simulink model "DCmotorArduinoUno"  (R2021b)
settings: Solver=FixedStepAuto  StartTime=0.0  StopTime=inf  FixedStep=.005  RelTol=1e-3  EnableMultiTasking=on
InitFcn:
  | pos = 0;
  | vel = 0;
model workspace: external: MATLAB File C:\My_Disk\work\school\grad\ME5245\finalProject\simulinkParameters.m (data not in the file)
values from neighbouring files (symbols this model uses):
  J = 0.018256    [simulinkParameters.m]
  Ts = 0.05    [simulinkParameters.m]
undefined symbols (not defined in the file or in its folder): DiscIntNeverNeededParam
libraries: arduinolib x8, fl_lib x5, nesl_utility x5, ee_lib x2, arduinosensorlib x1, slpidlib x1, simulink x1
settings Model: ExtModeTrigDuration=2  Creator=min  LastModifiedBy=min
settings SolverCC: PositivePriorityOrder=on  AutoInsertRateTranBlk=on  MinimalZcImpactIntegration=on
settings OptimizationCC: EnhancedBackFolding=on  PassReuseOutputArgsAs=Individual arguments  ZeroExternalMemoryAtStartup=off  ZeroInternalMemoryAtStartup=off  MaxStackSize=64  OptimizeBlockOrder=speed  DifferentSizesBufferReuse=on  OptimizationCustomize=off  EfficientTunableParamExpr=on
settings DebuggingCC: ReadBeforeWriteMsg=DisableAll  WriteAfterWriteMsg=DisableAll  WriteAfterReadMsg=DisableAll  TasksWithSamePriorityMsg=none  ParameterTunabilityLossMsg=error
settings HardwareCC: ProdBitPerInt=16  ProdBitPerPointer=16  ProdBitPerSizeT=16  ProdBitPerPtrDiffT=16  ProdLargestAtomicFloat=None  ProdWordSize=8  ProdHWDeviceType=Atmel->AVR  UseEmbeddedCoderFeatures=off
settings ModelReferenceCC: UpdateModelReferenceTargets=IfOutOfDate
settings SFSimCC: SFSimEcho=off  MATLABDynamicMemAlloc=off
settings RTWCC: Description=Embedded Coder  SystemTargetFile=ert.tlc  HardwareBoard=Arduino Uno  TemplateMakefile=ert_default_tmf  Toolchain=Arduino AVR  BuildConfiguration=Faster Runs  CodeExecutionProfiling=on  TargetLang=C++
settings CodeAppCC: ForceParamTrailComments=on  IgnoreCustomStorageClasses=off  OperatorAnnotations=on  SimulinkDataObjDesc=on  SFDataObjDesc=on  InsertBlockDesc=on
settings ERTTargetCC: CodeInterfacePackaging=C++ class  SupportContinuousTime=on  SupportNonInlinedSFcns=on  SupportVariableSizeSignals=on  ExtModeTransport=3  ExtModeStaticAlloc=on  ExtModeStaticAllocSize=250  ExtModeMexFile=ext_xcp  ExtModeIntrfLevel=Level2 - Open  RootIOFormat=Structure reference

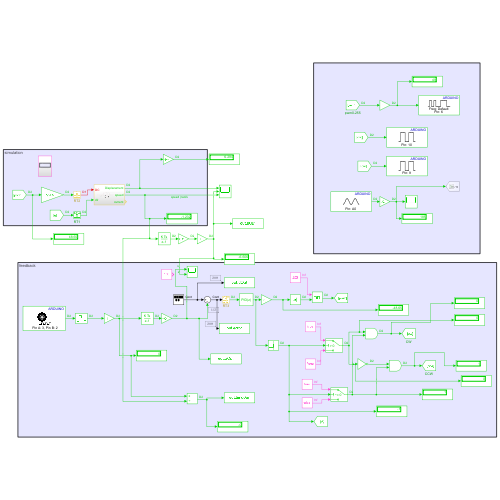
[thumbnail: Simulink's stored preview of the top-level diagram]
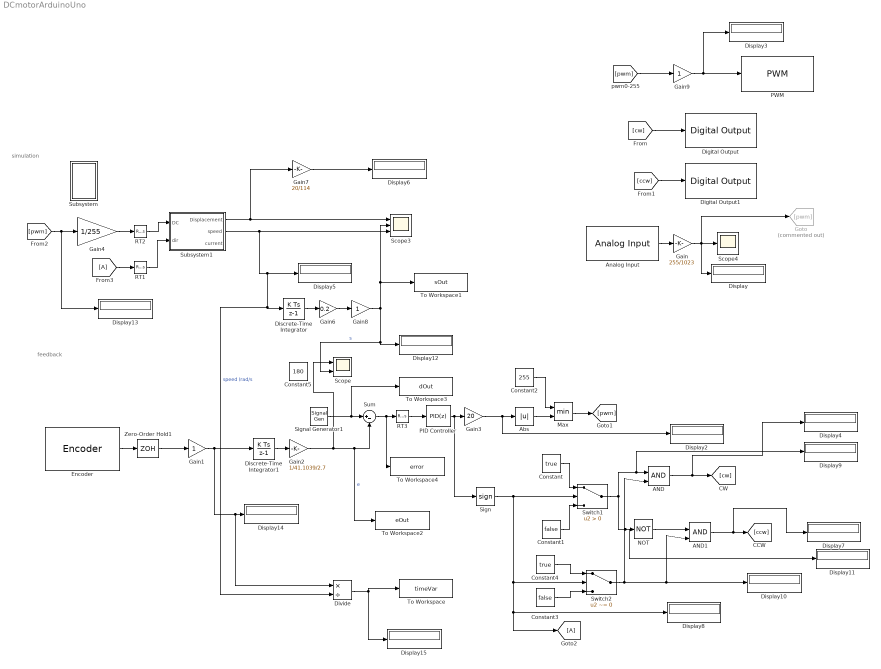
== system DCmotorArduinoUno ==
  note: feedback
  note: simulation
  AND : Logic  IconShape=distinctive  AllPortsSameDT=off  OutDataTypeStr=boolean
  AND1 : Logic  IconShape=distinctive  AllPortsSameDT=off  OutDataTypeStr=boolean
  Abs : Abs
  Analog Input : arduinolib/Analog Input  pinNumber=0  ReadResultsOnly=off  ConversionTriggerSource=Software  ExternalTriggerType=uint32( 0 )  OutputDataType=uint16  EnableConversionCompleteNotify=off  EnableOuputStatus=off  SampleTime=Ts  blockPlatform=arduino
  Constant : Constant  Value=true
  Constant1 : Constant  Value=false
  Constant2 : Constant  Value=255
  Constant3 : Constant  Value=false
  Constant4 : Constant  Value=true
  Constant5 : Constant  Value=180
  Digital Output : arduinolib/Digital Output  pinNumber=driverIn1pin  Direction=output  blockPlatform=arduino
  Digital Output1 : arduinolib/Digital Output  pinNumber=driverIn2pin  Direction=output  blockPlatform=arduino
  Discrete-Time Integrator : DiscreteIntegrator  SampleTime=-1  ICPrevOutput=DiscIntNeverNeededParam  ICPrevScaledInput=DiscIntNeverNeededParam
  Discrete-Time Integrator1 : DiscreteIntegrator  SampleTime=-1  ICPrevOutput=DiscIntNeverNeededParam  ICPrevScaledInput=DiscIntNeverNeededParam
  Display{,2..15} (15 alike) : Display
  Divide : Product  Inputs=*/
  Encoder : arduinosensorlib/Encoder  InputA=3  InputB=2  Mode=Reset at each Sample time  SampleTime=Ts
      settings: SourceProductBaseCode=ARDUINO
  Gain : Gain  Gain=255/1023  OutDataTypeStr=uint8  RndMeth=Nearest
  Gain1 : Gain  OutDataTypeStr=int32
  Gain2 : Gain  Gain=1/41.1039/2.7
  Gain3 : Gain  Gain=20
  Gain4 : Gain  Gain=1/255  OutDataTypeStr=double
  Gain6 : Gain  Gain=0.2
  Gain7 : Gain  Gain=20/114
  Gain8 : Gain
  Gain9 : Gain  OutDataTypeStr=uint8  RndMeth=Nearest
  Goto : Goto  Commented=on  GotoTag=pwm
  Max : MinMax  Inputs=2
  NOT : Logic  Operator=NOT  IconShape=distinctive  AllPortsSameDT=off  OutDataTypeStr=boolean
  PID Controller : slpidlib/PID Controller  Controller=PID  Form=Parallel  TimeDomain=Discrete-time  UseExternalTs=off  SampleTime=-1  IntegratorMethod=Forward Euler  FilterMethod=Forward Euler  ControllerParametersSource=internal  P=.12  I=.71  D=0  UseFilter=on  N=100  TunerSelectOption=Transfer Function Based (PID Tuner App)  InitialConditionSource=internal  InitialConditionForIntegrator=0  InitialConditionForFilter=0  DifferentiatorICPrevScaledInput=0  ExternalReset=none  TrackingMode=off  Kt=1  LimitOutput=off  SatLimitsSource=internal  UpperSaturationLimit=inf  LowerSaturationLimit=-inf  LinearizeAsGain=on  AntiWindupMode=none  Kb=1  POutMin=[]  POutMax=[]  IOutMin=[]  IOutMax=[]  DOutMin=[]  DOutMax=[]  NOutMin=[]  NOutMax=[]  SumOutMin=[]  SumOutMax=[]  SaturationOutMin=[]  SaturationOutMax=[]  PParamMin=[]  PParamMax=[]  IParamMin=[]  IParamMax=[]  DParamMin=[]  DParamMax=[]  NParamMin=[]  NParamMax=[]  KbParamMin=[]  KbParamMax=[]  KtParamMin=[]  KtParamMax=[]  KbOutMin=[]  KbOutMax=[]  KtOutMin=[]  KtOutMax=[]  IntegratorOutMin=[]  IntegratorOutMax=[]  FilterOutMin=[]  FilterOutMax=[]  SumI1OutMin=[]  SumI1OutMax=[]  SumI2OutMin=[]  SumI2OutMax=[]  SumI3OutMin=[]  SumI3OutMax=[]  SumI4OutMin=[]  SumI4OutMax=[]  SumDOutMin=[]  SumDOutMax=[]  DifferentiatorOutMin=[]  DifferentiatorOutMax=[]  FilterDiffOutCoefMin=[]  FilterDiffOutCoefMax=[]  ReciprocalOutMin=[]  ReciprocalOutMax=[]  SumDenOutMin=[]  SumDenOutMax=[]  SumNumOutMin=[]  SumNumOutMax=[]  DivideOutMin=[]  DivideOutMax=[]  UdiffTsProdOutMin=[]  UdiffTsProdOutMax=[]  NTsProdOutMin=[]  NTsProdOutMax=[]  UintegralTsProdOutMin=[]  UintegralTsProdOutMax=[]  UngainTsProdOutMin=[]  UngainTsProdOutMax=[]  IntegratorContinuousStateAttributes=''  IntegratorStateMustResolveToSignalObject=off  IntegratorRTWStateStorageClass=Auto  FilterContinuousStateAttributes=''  FilterStateMustResolveToSignalObject=off  FilterRTWStateStorageClass=Auto  ParallelPVariant=InternalParameters  IdealPVariant=Disabled  IVariant=InternalParameters  DVariant=InternalParameters  IntegratorVariant=Discrete  SatVariant=Disabled  AWVariant=Passthrough  PCopyVariant=Disabled  TRVariant=Disabled  FdbkBlocksVariant=Forward  IdealPFdbkVariant=Disabled  SatFdbkVariant=Disabled  DerivativeFilterVariant=ForwardEulerFilter  NVariant=InternalParameters  NCopyVariant=Disabled  FilterICVariant=InternalICsFilter  IntegratorICVariant=InternalICs  ExternalResetVariant=Disabled  TRSumVariant=Passthrough  SumFdbkVariant=Disabled  SumVariant=Sum_PID  TsampFilterVariant=InternalTs  TsampNgainVariant=Passthrough  TsampIntegralVariant=Passthrough  ExternalSaturationOutDataTypeStr=Inherit: Same as second input
  PWM : arduinolib/PWM  pinNumber=6  frequencyType=Default  desiredFrequency=490.2  achievableFrequency=490.2
  RT1 : RateTransition  OutPortSampleTime=Ts
  RT2 : RateTransition  OutPortSampleTime=5e-3
  RT3 : RateTransition  OutPortSampleTime=Ts
  Scope : Scope  NumInputPorts=2
  Scope3 : Scope  NumInputPorts=3
  Scope4 : Scope
  Sign : Signum
  Signal Generator1 : SignalGenerator  WaveForm=square  Amplitude=pi/2  Frequency=.1
  Subsystem : Subsystem
  Subsystem1 : Subsystem
  Sum : Sum  Inputs=|+-
  Switch1 : Switch  Criteria=u2 > Threshold
  Switch2 : Switch  Criteria=u2 ~= 0
  To Workspace : ToWorkspace  VariableName=timeVar  SaveFormat=Timeseries  SampleTime=-1
  To Workspace1 : ToWorkspace  VariableName=sOut  SaveFormat=Timeseries  SampleTime=-1
  To Workspace2 : ToWorkspace  VariableName=eOut  SaveFormat=Timeseries  SampleTime=-1
  To Workspace3 : ToWorkspace  VariableName=dOut  SaveFormat=Timeseries  SampleTime=Ts
  To Workspace4 : ToWorkspace  VariableName=error  SaveFormat=Timeseries  SampleTime=Ts
  Zero-Order Hold1 : ZeroOrderHold  SampleTime=Ts
  wires:
  Analog Input/1 -> Gain/1
  Encoder/1 -> Zero-Order Hold1/1
  Zero-Order Hold1/1 -> Gain1/1
  Gain1/1 -> Discrete-Time Integrator1/1, Divide/1, Display14/1
  Gain/1 -> Display/1, Scope4/1, Goto/1
  Subsystem1/2(speed) -> Scope3/3, Divide/2, Discrete-Time Integrator/1, Display5/1  "speed (rad/s"
  RT2/1 -> Subsystem1/1(DC)
  Gain4/1 -> RT2/1
  Switch1/1 -> Display11/1, NOT/1, Display9/1, AND/1
  Constant1/1 -> Switch1/3
  Constant/1 -> Switch1/1
  Sign/1 -> Switch2/2, [A], Display8/1, Switch1/2
  Signal Generator1/1 -> To Workspace3/1, Sum/1
  Max/1 -> [pwm]
  Constant2/1 -> Max/1
  Abs/1 -> Max/2
  Switch2/1 -> AND1/2, Display10/1, AND/2
  AND/1 -> Display4/1, [cw]
  NOT/1 -> AND1/1
  AND1/1 -> Display7/1, [ccw]
  Gain3/1 -> Display2/1, Abs/1
  Constant4/1 -> Switch2/1
  Constant3/1 -> Switch2/3
  Subsystem1/1(Displacement) -> Gain7/1, Scope3/1
  Discrete-Time Integrator/1 -> Gain6/1
  [A] -> RT1/1
  Gain6/1 -> Gain8/1
  Gain7/1 -> Display6/1
  Gain8/1 -> Scope/2, Display12/1, To Workspace1/1, Scope3/2  "s"
  RT1/1 -> Subsystem1/2(dir)
  RT3/1 -> PID Controller/1
  Sum/1 -> To Workspace4/1, RT3/1
  PID Controller/1 -> Gain3/1, Sign/1
  Gain9/1 -> Display3/1, PWM/1
  [pwm] -> Gain9/1
  [cw] -> Digital Output/1
  Divide/1 -> Display15/1, To Workspace/1
  [pwm] -> Display13/1, Gain4/1
  Discrete-Time Integrator1/1 -> Gain2/1
  Gain2/1 -> To Workspace2/1, Sum/2, Scope/1  "e"
  [ccw] -> Digital Output1/1

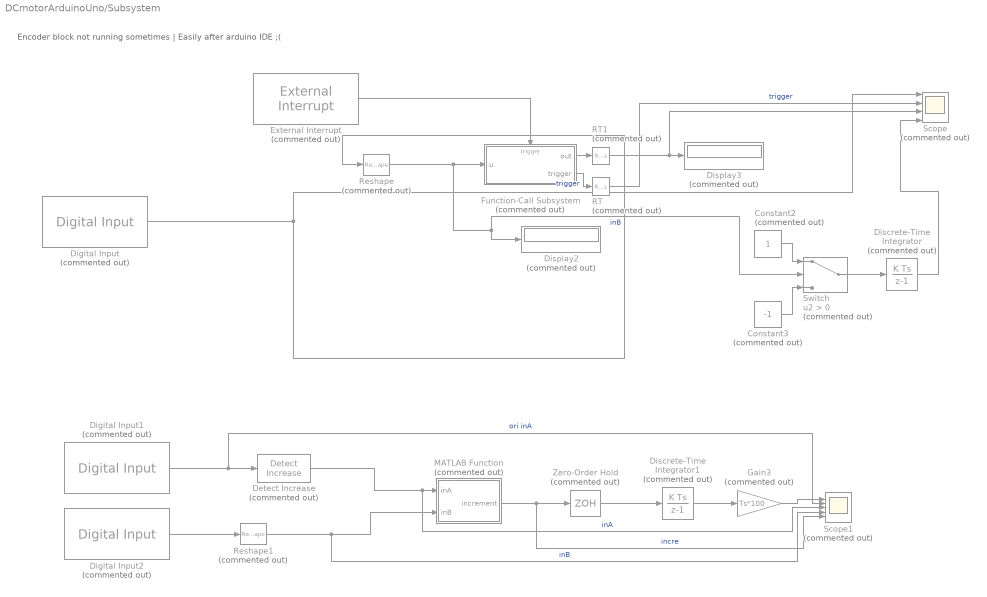
== system DCmotorArduinoUno/Subsystem ==
  note: Encoder block not running sometimes | Easily after arduino IDE ;(
  Constant2 : Constant  Commented=on
  Constant3 : Constant  Commented=on  Value=-1
  Detect Increase : simulink/Logic and Bit Operations/Detect Increase  Commented=on  vinit=0.0  OutDataTypeStr=boolean
  Digital Input : arduinolib/Digital Input  Commented=on  pinNumber=2  mode=Default  Direction=input  SampleTime=Ts  blockPlatform=arduino
  Digital Input1 : arduinolib/Digital Input  Commented=on  pinNumber=3  mode=Default  Direction=input  SampleTime=-1  blockPlatform=arduino
  Digital Input2 : arduinolib/Digital Input  Commented=on  pinNumber=2  mode=Default  Direction=input  SampleTime=Ts  blockPlatform=arduino
  Discrete-Time Integrator : DiscreteIntegrator  Commented=on  gainval=100  SampleTime=Ts  ICPrevOutput=DiscIntNeverNeededParam  ICPrevScaledInput=DiscIntNeverNeededParam
  Discrete-Time Integrator1 : DiscreteIntegrator  Commented=on  SampleTime=-1  ICPrevOutput=DiscIntNeverNeededParam  ICPrevScaledInput=DiscIntNeverNeededParam
  Display2 : Display  Commented=on
  Display3 : Display  Commented=on
  External Interrupt : arduinolib/External Interrupt  Commented=on  Pin=3  PullUp=off  Mode=RISING  InterruptSimulationInput=off
      settings: SourceProductBaseCode=ARDUINO
  Function-Call Subsystem : Subsystem  Commented=on  InitFcn=|  TreatAsAtomicUnit=on  mask{pos=pos, vel=vel}
      | pos = 0;
      | vel = 0;
      mask prompts: pos "Global Pos var"; vel "Global Vel var"
  Gain3 : Gain  Commented=on  Gain=Ts*100
  MATLAB Function : MATLAB Function  Commented=on  TreatAsAtomicUnit=on
  RT : RateTransition  Commented=on  Deterministic=off
  RT1 : RateTransition  Commented=on  Deterministic=off
  Reshape : Reshape  Commented=on
  Reshape1 : Reshape  Commented=on
  Scope : Scope  Commented=on  NumInputPorts=4
  Scope1 : Scope  Commented=on  NumInputPorts=5
  Switch : Switch  Commented=on  Criteria=u2 > Threshold
  Zero-Order Hold : ZeroOrderHold  Commented=on  SampleTime=-1
  wires:
  RT1/1 -> Display3/1, Scope/3
  Digital Input/1 -> Scope/1, Reshape/1
  Gain3/1 -> Scope1/1
  Constant2/1 -> Switch/1
  Digital Input1/1 -> Scope1/2, Detect Increase/1  "ori inA"
  Reshape/1 -> Switch/2, Display2/1, Function-Call Subsystem/1(u)  "inB"
  Zero-Order Hold/1 -> Discrete-Time Integrator1/1
  Discrete-Time Integrator1/1 -> Gain3/1
  Function-Call Subsystem/2(trigger) -> RT/1  "trigger"
  Constant3/1 -> Switch/3
  RT/1 -> Scope/2  "trigger"
  MATLAB Function/1(increment) -> Scope1/5, Zero-Order Hold/1  "incre"
  Detect Increase/1 -> Scope1/3, MATLAB Function/1(inA)  "inA"
  Function-Call Subsystem/1(out) -> RT1/1
  Discrete-Time Integrator/1 -> Scope/4
  Digital Input2/1 -> Reshape1/1
  Switch/1 -> Discrete-Time Integrator/1
  External Interrupt/1 -> Function-Call Subsystem/Trigger
  Reshape1/1 -> Scope1/4, MATLAB Function/2(inB)  "inB"

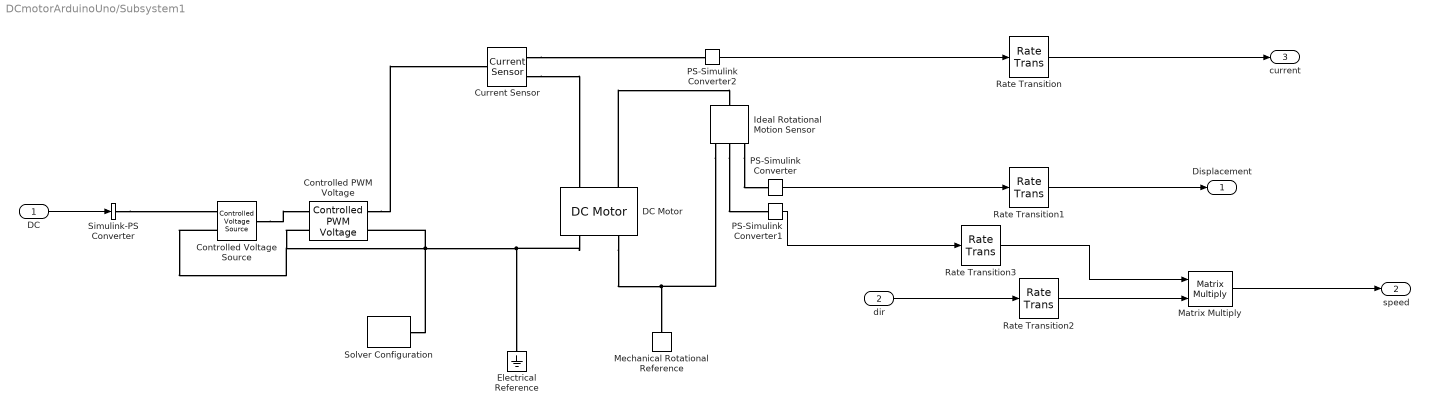
== system DCmotorArduinoUno/Subsystem1 ==
  DC : Inport
  dir : Inport  Port=2
  Controlled PWM Voltage : ee_lib/Integrated Circuits/Controlled PWM Voltage  F=100 Hz  TD=0 s  pulse_width_offset=0 s  pulse_min=0 s  pwm_or_av=1  event_type=1  sample_time=1e-6 s  Vmin=0 V  Vmax=1 V  Vm=6 V  u_min=0  u_max=1
  Controlled Voltage Source : fl_lib/Electrical/Electrical Sources/Controlled Voltage Source
  Current Sensor : fl_lib/Electrical/Electrical Sensors/Current Sensor
  DC Motor : ee_lib/Electromechanical/Brushed Motors/DC Motor  field_option=ee.enum.field_option.pm  Rf=100 Ohm  Lf=1 H  Laf=0.15 H  If0=0 A  parameterization=ee.enum.dcparam_option.circuit_param  Ra=R Ohm  La=L H  emf_or_torque=ee.enum.emf_or_torque.kv  Kv=kb V/(rad/s)  Ki=6.876e-4 N*m/A  T_stall=0.24e-3 N*m  w_max=19100 rpm  w_rated=15000 rpm  P_rated=0.08 W  V_rated=1.5 V  lam_param=ee.enum.lam_param.damping  i_noload=0 A  V_i_noload=1.5 V  J=J kg*m^2  lam=b N*m/(rad/s)  speed0=0 rpm  enable_fault_armature=simscape.enum.onoff.off  rev_faulted=1 / 3  G_faulted_armature=1e-5 S  fault_trigger_armature=ee.enum.faults.faultTrigger.temporal  t_fault_armature=1 s  max_permissible_current_armature=inf A  t_fail_on_current_armature=1 s  enable_fault_field=simscape.enum.onoff.off  G_faulted_field=1e-5 S  fault_trigger_field=ee.enum.faults.faultTrigger.temporal  t_fault_field=1 s  max_permissible_current_field=inf A  t_fail_on_current_field=1 s  fault_action=simscape.enum.assert.action.none  alpha=3.93e-3 1/K  Tmeas=25 degC  thermal_mass=100 J/K  initial_temperature=25 degC
  Electrical Reference : fl_lib/Electrical/Electrical Elements/Electrical Reference
  Ideal Rotational Motion Sensor : fl_lib/Mechanical/Mechanical Sensors/Ideal Rotational Motion Sensor  wrap_angle=simscape.enum.onoff.off  offset=0 rad
  Matrix Multiply : Product  Multiplication=Matrix(*)
  Mechanical Rotational Reference : fl_lib/Mechanical/Rotational Elements/Mechanical Rotational Reference
  PS-Simulink Converter : nesl_utility/PS-Simulink Converter  PhysicalDomain=network_engine_domain  SubClassName=ps_output  LeftPortType=input  RightPortType=output  PseudoPeriodic=off  Frequencies=[]  Unit=inherit  AffineConversion=off
      settings: SourceProductBaseCode=PW,SS
  PS-Simulink Converter1 : nesl_utility/PS-Simulink Converter  PhysicalDomain=network_engine_domain  SubClassName=ps_output  LeftPortType=input  RightPortType=output  PseudoPeriodic=off  Frequencies=[]  Unit=inherit  AffineConversion=off
      settings: SourceProductBaseCode=PW,SS
  PS-Simulink Converter2 : nesl_utility/PS-Simulink Converter  PhysicalDomain=network_engine_domain  SubClassName=ps_output  LeftPortType=input  RightPortType=output  PseudoPeriodic=off  Frequencies=[]  Unit=inherit  AffineConversion=off
      settings: SourceProductBaseCode=PW,SS
  Rate Transition{,1..3} (4 alike) : RateTransition  OutPortSampleTime=Ts
  Simulink-PS Converter : nesl_utility/Simulink-PS Converter  PhysicalDomain=network_engine_domain  SubClassName=ps_input  LeftPortType=input  RightPortType=output  PseudoPeriodic=off  Frequencies=[]  NoiseDistribution=none  NoiseParameters=[]  Unit=1  AffineConversion=off  FilteringAndDerivatives=provide  SimscapeFilterOrder=1  InputFilterTimeConstant=0.001  UdotUserProvided=0
      settings: SourceProductBaseCode=PW,SS
  Solver Configuration : nesl_utility/Solver Configuration  PhysicalDomain=network_engine_domain  SubClassName=solver  LeftPortType=input  RightPortType=generic  Tones=[]  Harmonics=[]  SimulateNoise=off  Profile=off  UseLocalSampling=off  EnableSwitchedLinearOptims=on  FrequencyDomain=off  UseCCode=off  RelTol=0.001  AbsTol=1e-06  MinStep=1e-09  ToWorkspace=off  RevertToSquareIcSolve=off  NumHomotopyIterations=100  PhasorMode=off  PhasorModeNumHarmonics=1  DoDC=off  ResidualTolerance=1e-09  UseLocalSolver=off  LocalSolverChoice=NE_BACKWARD_EULER_ADVANCER  LocalSolverSampleTime=0.001  DoFixedCost=off  MaxNonlinIter=3  MaxModeIter=2  ComputeImpulses=off  ImpulseIterations=2  LinearAlgebra=auto  EquationFormulation=NE_TIME_EF  DelaysMemoryBudget=1024  AutomaticFiltering=on  FilteringTimeConstant=0.001  PartitionStorageMethod=AS_NEEDED  PartitionMemoryBudget=1024  PartitionMethod=ROBUST
      settings: SourceProductBaseCode=PW,SS
  Displacement : Outport
  speed : Outport  Port=2
  current : Outport  Port=3
  wires:
  PS-Simulink Converter2/1 -> Rate Transition/1
  DC/1 -> Simulink-PS Converter/1
  dir/1 -> Rate Transition2/1
  PS-Simulink Converter1/1 -> Rate Transition3/1
  Matrix Multiply/1 -> speed/1
  PS-Simulink Converter/1 -> Rate Transition1/1
  Rate Transition/1 -> current/1
  Rate Transition1/1 -> Displacement/1
  Rate Transition2/1 -> Matrix Multiply/2
  Rate Transition3/1 -> Matrix Multiply/1
  ? -> ?
  connections:
  DC Motor/LConn2 -- Ideal Rotational Motion Sensor/LConn1
  DC Motor/RConn2 -- Ideal Rotational Motion Sensor/RConn1 -- Mechanical Rotational Reference/LConn1
  Solver Configuration/RConn1 -- Controlled Voltage Source/RConn2 -- Controlled PWM Voltage/LConn2 -- Controlled PWM Voltage/RConn2 -- DC Motor/RConn1 -- Electrical Reference/LConn1
  Controlled PWM Voltage/RConn1 -- Current Sensor/LConn1
  Current Sensor/RConn2 -- DC Motor/LConn1
  Ideal Rotational Motion Sensor/RConn3 -- PS-Simulink Converter/LConn1
  Ideal Rotational Motion Sensor/RConn2 -- PS-Simulink Converter1/LConn1
  Current Sensor/RConn1 -- PS-Simulink Converter2/LConn1
  Simulink-PS Converter/RConn1 -- Controlled Voltage Source/RConn1
  Controlled Voltage Source/LConn1 -- Controlled PWM Voltage/LConn1

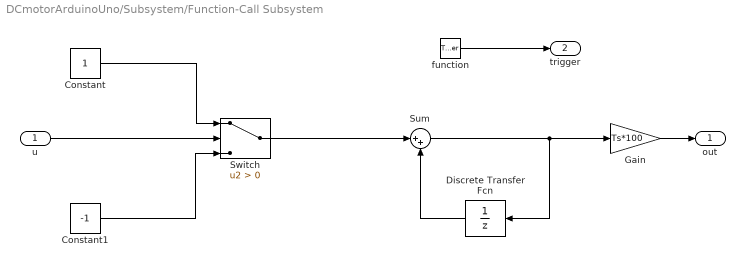
== system DCmotorArduinoUno/Subsystem/Function-Call Subsystem ==
  u : Inport
  function : TriggerPort  TriggerType=function-call  VariantControl=(inherit)  ShowOutputPort=on
  Constant : Constant
  Constant1 : Constant  Value=-1
  Discrete Transfer Fcn : DiscreteTransferFcn  Denominator=[1 0]
  Gain : Gain  Gain=Ts*100
  Sum : Sum  Inputs=|++
  Switch : Switch  Criteria=u2 > Threshold
  out : Outport
  trigger : Outport  Port=2
  wires:
  u/1 -> Switch/2
  Constant/1 -> Switch/1
  Constant1/1 -> Switch/3
  Gain/1 -> out/1
  Discrete Transfer Fcn/1 -> Sum/2
  Sum/1 -> Discrete Transfer Fcn/1, Gain/1
  Switch/1 -> Sum/1
  function/1 -> trigger/1

== matlab function DCmotorArduinoUno/Subsystem/MATLAB Function ==
  data: inA input; increment output; inB input
function increment = fcn(inA,inB)
if inA
    if inB
        increment = 1;
    else
        increment = -1;
    end
else
    increment = 0;
end
end
